simulink model "One_ZRM_MFKT"  (R2016a)
settings: Solver=VariableStepAuto  StartTime=0.0  StopTime=10.0  RelTol=1e-3
values from neighbouring files (symbols this model uses):
  T_z_AP = 0    [Computation_Reduced_Model.m]    (also in Untitled.m)
  x_AP = [0;0;0]    [Computation_Reduced_Model.m]    (also in One_ZRM.m = [0;0;0;0;0;0]; Untitled.m)
libraries: simulink x1
settings Model: Creator=Florian  LastModifiedBy=Florian

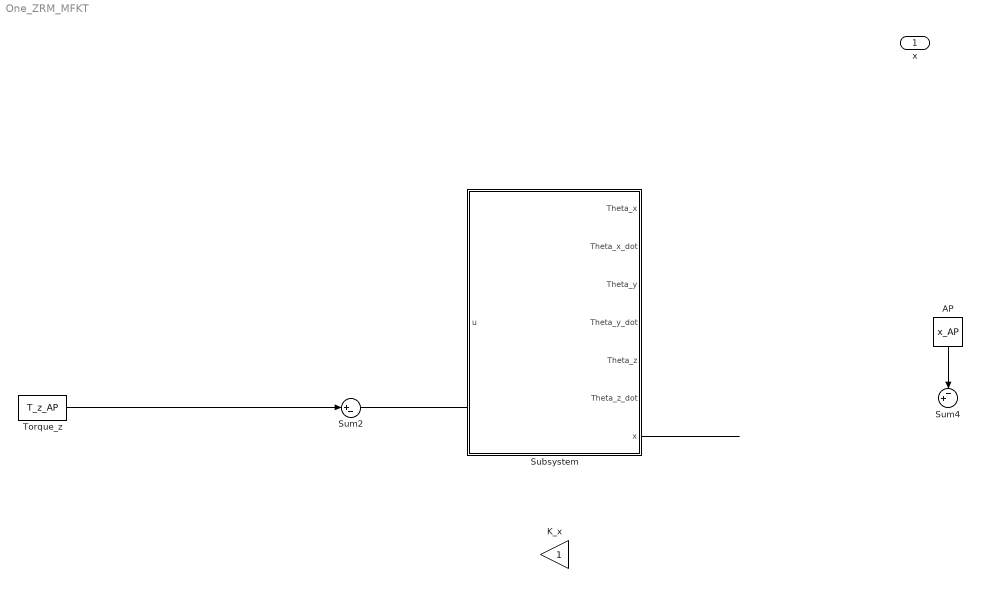
== system One_ZRM_MFKT ==
  "AP " : Constant  Value=x_AP
  K_x : Gain
  Subsystem : Subsystem
  Sum2 : Sum  Inputs=|+-
  Sum4 : Sum  Inputs=-+|
  Torque_z : Constant  Value=T_z_AP
  x : Outport
  wires:
  Sum2/1 -> ?
  Torque_z/1 -> Sum2/1
  Subsystem/7(x) -> ?
  "AP "/1 -> Sum4/1

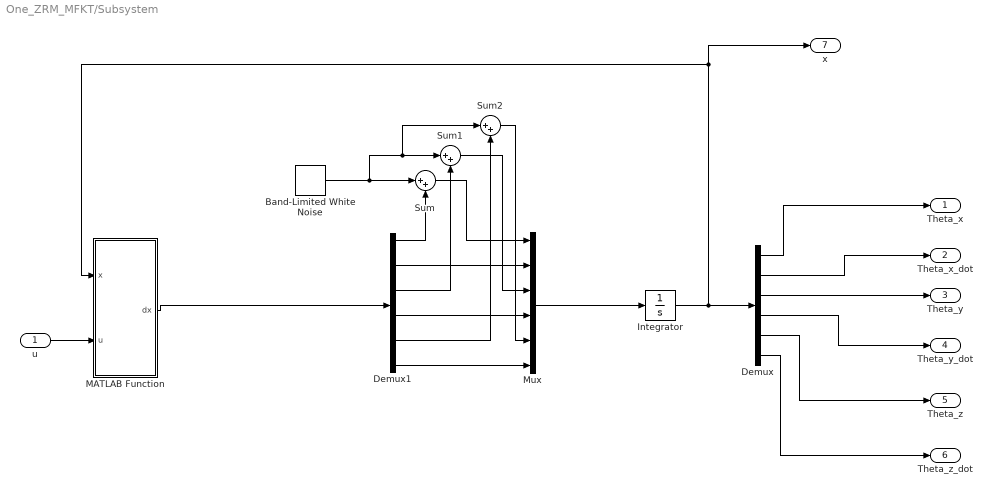
== system One_ZRM_MFKT/Subsystem ==
  "u " : Inport
  Band-Limited White Noise : simulink/Sources/Band-Limited White Noise  Cov=[0.1^2]  Ts=1/92  seed=[23341]
  Demux : Demux  Outputs=6
  Demux1 : Demux  Outputs=6
  Integrator : Integrator  InitialCondition="[0 pi/32  0 0]"
  MATLAB Function : MATLAB Function  TreatAsAtomicUnit=on
  Mux : Mux  Inputs=6
  Sum : Sum  Inputs=|++
  Sum1 : Sum  Inputs=|++
  Sum2 : Sum  Inputs=|++
  Theta_x : Outport
  Theta_x_dot : Outport  Port=2
  Theta_y : Outport  Port=3
  Theta_y_dot : Outport  Port=4
  Theta_z : Outport  Port=5
  Theta_z_dot : Outport  Port=6
  x : Outport  Port=7
  wires:
  MATLAB Function/1(dx) -> Demux1/1
  Band-Limited White Noise/1 -> Sum2/1, Sum1/1, Sum/1
  Integrator/1 -> Demux/1, x/1, MATLAB Function/1(x)
  Demux1/6 -> Mux/6
  Sum/1 -> Mux/1
  Demux1/3 -> Sum1/2
  Demux1/5 -> Sum2/2
  Mux/1 -> Integrator/1
  Demux1/1 -> Sum/2
  Sum1/1 -> Mux/3
  Demux1/4 -> Mux/4
  Demux1/2 -> Mux/2
  Sum2/1 -> Mux/5
  Demux/3 -> Theta_y/1
  Demux/1 -> Theta_x/1
  Demux/5 -> Theta_z/1
  Demux/2 -> Theta_x_dot/1
  Demux/4 -> Theta_y_dot/1
  Demux/6 -> Theta_z_dot/1
  "u "/1 -> MATLAB Function/2(u)

== matlab function One_ZRM_MFKT/Subsystem/MATLAB Function ==
  data: x input; dx output; u input
function dx = fcn(x,u)

T_x = u(1);
T_y = u(2);
T_z = u(3);

theta_x = x(1);
theta_x_dot = x(2);
theta_y = x(3);
theta_y_dot = x(4);
theta_z = x(5);
theta_z_dot = x(6); 

theta_x_dotdot = f_yz; 
theta_y_dotdot = f_xz; 
theta_z_dotdot = f_xy; 



dx = [theta_x_dot, theta_x_dotdot, theta_y_dot, theta_y_dotdot, theta_z_dot, theta_z_dotdot];
